simulink model "Series_RLC_System"  (R2022b)
settings: Solver=FixedStepAuto  StartTime=0.0  StopTime=10.0  FixedStep=1e-3  RelTol=1e-3
settings Model: Creator=MAAM  LastModifiedBy=MAAM

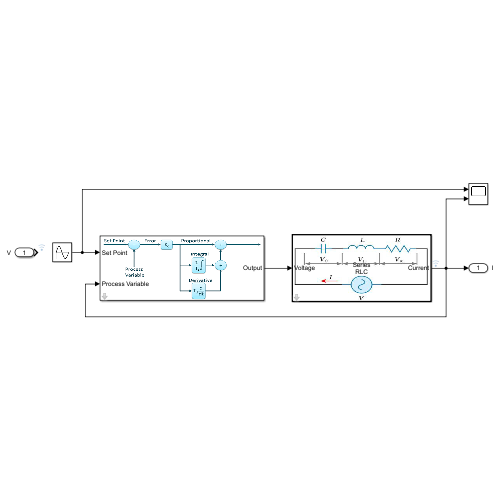
[thumbnail: Simulink's stored preview of the top-level diagram]
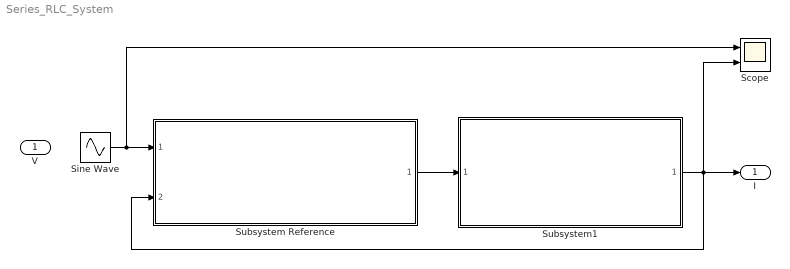
== system Series_RLC_System ==
  V : Inport
  Scope : Scope  NumInputPorts=2
  Sine Wave : Sin  SampleTime=0
  Subsystem Reference : Subsystem  ReferencedSubsystem=PID_Ideal  Kp=10  Ki=0.01  Kd=100e-6
  Subsystem1 : Subsystem  TreatAsAtomicUnit=on  ReferencedSubsystem=RLC_Series  R=10  L=0.01  C=100e-6
  I : Outport
  wires:
  Sine Wave/1 -> Scope/1, Subsystem Reference/1
  Subsystem1/1 -> Scope/2, Subsystem Reference/2, I/1
  Subsystem Reference/1 -> Subsystem1/1
